simulink subsystem "thermostatController"  (R2023a)
settings: Solver=VariableStepAuto  StartTime=0.0  StopTime=10.0  RelTol=1e-3
InitFcn:
  | setupPID
undefined symbols (not defined in the file): integral, proportional
settings Model: DefaultTestHarness=thermostatController_SimHarness  Creator=Sam  LastModifiedBy=Sam

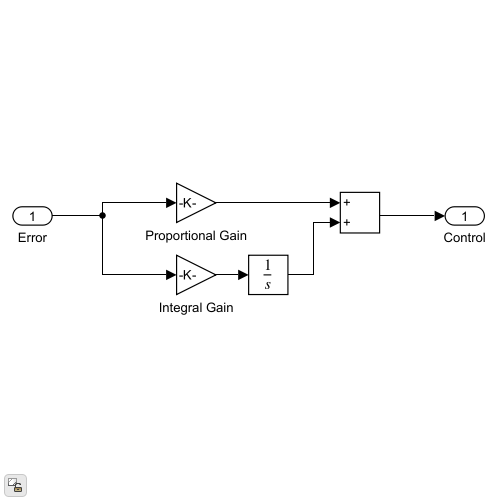
[thumbnail: Simulink's stored preview of the top-level diagram]
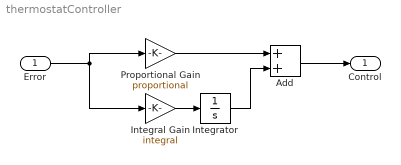
== system thermostatController ==
  Error : Inport
  Add : Sum
  Integral Gain : Gain  Gain=integral
  Integrator : Integrator
  Proportional Gain : Gain  Gain=proportional
  Control : Outport
  wires:
  Error/1 -> Proportional Gain/1, Integral Gain/1
  Add/1 -> Control/1
  Integral Gain/1 -> Integrator/1
  Proportional Gain/1 -> Add/1
  Integrator/1 -> Add/2
